simulink model "DigitalTwinMachine"  (R2023b)
settings: Solver=FixedStepAuto  StartTime=0.0  StopTime=0.2  FixedStep=0.001  RelTol=1e-1
undefined symbols (not defined in the file or in its folder): gray
libraries: fl_lib x40, nesl_utility x13, ee_lib x6, batteryecm_lib x1
settings Model: PacingRate=0.022000  Creator=Utente  LastModifiedBy=Utente
settings OptimizationCC: ReuseModelBlockBuffer=off
settings DebuggingCC: ParameterOverflowMsg=none
settings SFSimCC: SimTargetLang=C++

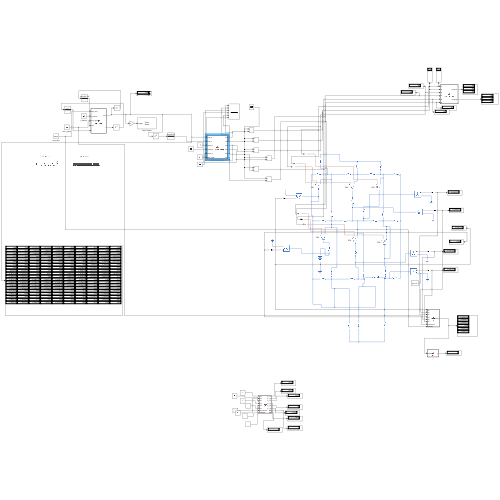
[thumbnail: Simulink's stored preview of the top-level diagram]
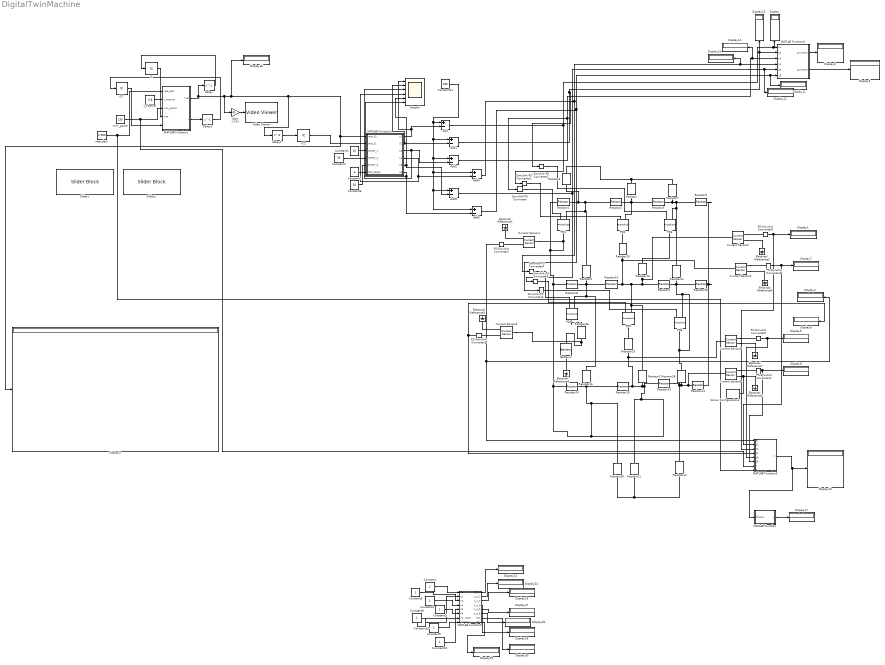
== system DigitalTwinMachine ==
  Add{,1..5} (6 alike) : Sum  Inputs=+-
  Battery1 : batteryecm_lib/Battery  Vnom=12 V  prm_dir=simscape.enum.battery.prm_dir.disabled  R1_dis=2 Ohm  R1_ch=2 Ohm  R1=2 Ohm  prm_AH=simscape.enum.battery.prm_AH.infinite  AH=50 A*hr  V1=11.5 V  AH1=25 A*hr  prm_R2=simscape.enum.battery.prm_R2.disabled  R2=2000 Ohm  Tmeas=298.15 K  charge_measurement_port=simscape.enum.battery.enable.no  prm_dyn=simscape.enum.battery.prm_dyn.off  Rp1=0.005 Ohm  tau1=30 s  Rp2=0.005 Ohm  tau2=30 s  Rp3=0.005 Ohm  tau3=30 s  Rp4=0.005 Ohm  tau4=30 s  Rp5=0.005 Ohm  tau5=30 s  prm_fade=simscape.enum.battery.prm_fade.disabled  N_fade=100  AH_fade=45 A*hr  R1_fade=2.02 Ohm  R1_ch_fade=2.02 Ohm  V1_fade=10.35 V  prm_age=simscape.enum.battery.prm_age.disabled  prm_age_OCV=simscape.enum.battery.prm_age_OCV.OCV  OCV_age=0.9  SOC_age=60  Tmeas_age=298.15 K  delta_time_age_vec=[0] d  temperature_age_vec=[273] K  OCV_scaling_age=2.2134e6  OCV_offset_age=1.632e6  temp_exp_age=0.515833569 V  t_exp_age=0.75  Vnom_T2=12 V  R1_T2=2.2 Ohm  R1_T2_dis=2.2 Ohm  R1_T2_ch=2.2 Ohm  V1_T2=11.4 V  R2_T2=2200 Ohm  Rp1_T2=0.005 Ohm  tau1_T2=30 s  Rp2_T2=0.005 Ohm  tau2_T2=30 s  Rp3_T2=0.005 Ohm  tau3_T2=30 s  Rp4_T2=0.005 Ohm  tau4_T2=30 s  Rp5_T2=0.005 Ohm  tau5_T2=30 s  Tmeas2=273.15 K  thermal_port=simscape.enum.thermaleffects.omit  thermal_mass=30000 J/K  i_specify=off  i_priority=None  i=0 A  i_nominal_specify=off  i_nominal_unit=A  i_nominal_value=1  v_specify=off  v_priority=None  v=0 V  v_nominal_specify=off  v_nominal_unit=V  v_nominal_value=1  charge_specify=off  charge_priority=High  charge=50 A*hr  charge_nominal_specify=off  charge_nominal_unit=A*hr  charge_nominal_value=1  num_cycles_specify=off  num_cycles_priority=High  num_cycles=0  num_cycles_nominal_specify=off  num_cycles_nominal_unit=1  num_cycles_nominal_value=1  temperature_specify=off  temperature_priority=High  temperature=298.15 K  temperature_nominal_specify=off  temperature_nominal_unit=K  temperature_nominal_value=1
  Constant{,3..5,8..10,12} (8 alike) : Constant
  Constant1 : Constant  Value=10
  Constant11 : Constant  Value=185
  Constant2 : Constant  Value=30
  Constant6 : Constant  Value=50
  Constant7 : Constant  Value=6
  Current Sensor{1..6} (6 alike) : fl_lib/Electrical/Electrical Sensors/Current Sensor
  Delay : Delay  DelayLength=1  InitialCondition=0
  Delay1 : Delay  DelayLength=1  InitialCondition=0
  Delay2 : Delay  InitialCondition=0
  Display{,1..17,23..30} (26 alike) : Display
  Electrical Reference{1..7} (7 alike) : fl_lib/Electrical/Electrical Elements/Electrical Reference
  Gain : Gain  Gain=1/255
  IC : InitialCondition  Value=zeros(100,100)
  IC1 : InitialCondition
  IC2 : InitialCondition  Value=zeros(100,100)
  MATLAB Function : MATLAB Function  TreatAsAtomicUnit=on
  MATLAB Function1 : MATLAB Function  TreatAsAtomicUnit=on
  MATLAB Function2 : MATLAB Function  TreatAsAtomicUnit=on
  MATLAB Function3 : MATLAB Function  TreatAsAtomicUnit=on
  MATLAB Function4 : MATLAB Function  TreatAsAtomicUnit=on
  MATLAB Function5 : MATLAB Function  TreatAsAtomicUnit=on
  PD1 : ee_lib/Sensors & Transducers/Photodiode  prmFlux=2  Imeas=25 uA  FluxD=5 W/m^2  G=5e-6 A*m^2/W  prmExp=1  I2=0.1 A  V2=1.3 V  IS=5e-9 A  ec=3  RS=0.1 Ohm  Tmeas=25 degC  C_param=1  CJ=60 pF  CJ0=60 pF  VJ=1 V  Mgrad=0.5  Vvec=[.1, 10, 100] V  Cvec=[45, 3, 6] pF  FC=0.5  T_param=1  IS_T2=2.5e-7 A  I1_T2=0.07 A  V1_T2=1.3 V  Tmeas2=125 degC  EG_param=1  EG=1.11 eV  XTI_param=1  XTI=3  Tdevice=25 degC  i_specify=off  i_priority=None  i=0 A  i_nominal_specify=off  i_nominal_unit=A  i_nominal_value=1  v_specify=off  v_priority=None  v=0 V  v_nominal_specify=off  v_nominal_unit=V  v_nominal_value=1  v_capacitor_specify=off  v_capacitor_priority=High  v_capacitor=0 V  v_capacitor_nominal_specify=off  v_capacitor_nominal_unit=V  v_capacitor_nominal_value=1  thermal_network_parameterization=ee.enum.thermalNetworkTopology.junctionCase  Rth=[0, 10] K/W  Rth_Cauer=[1, 3, 10] K/W  Rth_Foster=[4, 6] K/W  thermal_mass_parameterization=ee.enum.thermalNetwork.timeconstant  thermal_mass=[0, 1] J/K  thermal_mass_Cauer=[1.5, 2, 3] J/K  thermal_mass_Foster=[1.5, 3] J/K  thermal_time_constant=[0, 10] s  thermal_time_constant_Cauer=[1, 3, 10] s  thermal_time_constant_Foster=[6, 18] s  thermal_mass_initial_temperatures=[25, 25] degC  thermal_mass_initial_temperatures_Cauer=[25, 25, 25] degC  steadyState_Foster=simscape.enum.onoff.on  Tvec_initial_Foster=[25, 25, 25, 25] degC
      settings: InternalSimscapePortConfiguration="{\"Bottom\":[],\"Left\":[{\"id\":\"W\",\"label\":\"W\",\"type\":\"input\"},{\"id\":\"p\",\"label\":\"\",\"type\":\"foundation.electrical.electrical\"}],\"Right\":[{\"id\":\"n\",\"label\":\"\",\"type\":\"foundation.electrical.electrical\"}],\"Top\":[]}"
  PD{2..3,5..6} (4 alike) : ee_lib/Sensors & Transducers/Photodiode  prmFlux=1  Imeas=25 uA  FluxD=5 W/m^2  G=5e-6 A*m^2/W  prmExp=1  I2=0.1 A  V2=1.3 V  IS=5e-9 A  ec=3  RS=0.1 Ohm  Tmeas=25 degC  C_param=1  CJ=60 pF  CJ0=60 pF  VJ=1 V  Mgrad=0.5  Vvec=[.1, 10, 100] V  Cvec=[45, 3, 6] pF  FC=0.5  T_param=1  IS_T2=2.5e-7 A  I1_T2=0.07 A  V1_T2=1.3 V  Tmeas2=125 degC  EG_param=1  EG=1.11 eV  XTI_param=1  XTI=3  Tdevice=25 degC  i_specify=off  i_priority=None  i=0 A  i_nominal_specify=off  i_nominal_unit=A  i_nominal_value=1  v_specify=off  v_priority=None  v=0 V  v_nominal_specify=off  v_nominal_unit=V  v_nominal_value=1  v_capacitor_specify=off  v_capacitor_priority=High  v_capacitor=0 V  v_capacitor_nominal_specify=off  v_capacitor_nominal_unit=V  v_capacitor_nominal_value=1  thermal_network_parameterization=ee.enum.thermalNetworkTopology.junctionCase  Rth=[0, 10] K/W  Rth_Cauer=[1, 3, 10] K/W  Rth_Foster=[4, 6] K/W  thermal_mass_parameterization=ee.enum.thermalNetwork.timeconstant  thermal_mass=[0, 1] J/K  thermal_mass_Cauer=[1.5, 2, 3] J/K  thermal_mass_Foster=[1.5, 3] J/K  thermal_time_constant=[0, 10] s  thermal_time_constant_Cauer=[1, 3, 10] s  thermal_time_constant_Foster=[6, 18] s  thermal_mass_initial_temperatures=[25, 25] degC  thermal_mass_initial_temperatures_Cauer=[25, 25, 25] degC  steadyState_Foster=simscape.enum.onoff.on  Tvec_initial_Foster=[25, 25, 25, 25] degC
      settings: InternalSimscapePortConfiguration="{\"Bottom\":[],\"Left\":[{\"id\":\"W\",\"label\":\"W\",\"type\":\"input\"},{\"id\":\"p\",\"label\":\"\",\"type\":\"foundation.electrical.electrical\"}],\"Right\":[{\"id\":\"n\",\"label\":\"\",\"type\":\"foundation.electrical.electrical\"}],\"Top\":[]}"
  PD4 : ee_lib/Sensors & Transducers/Photodiode  prmFlux=1  Imeas=25 uA  FluxD=5 W/m^2  G=5e-6 A*m^2/W  prmExp=1  I2=1 A  V2=10 V  IS=5e-9 A  ec=3  RS=0.1 Ohm  Tmeas=25 degC  C_param=1  CJ=60 pF  CJ0=60 pF  VJ=1 V  Mgrad=0.5  Vvec=[.1, 10, 100] V  Cvec=[45, 3, 6] pF  FC=0.5  T_param=1  IS_T2=2.5e-7 A  I1_T2=0.07 A  V1_T2=1.3 V  Tmeas2=125 degC  EG_param=1  EG=1.11 eV  XTI_param=1  XTI=3  Tdevice=25 degC  i_specify=off  i_priority=None  i=0 A  i_nominal_specify=off  i_nominal_unit=A  i_nominal_value=1  v_specify=off  v_priority=None  v=0 V  v_nominal_specify=off  v_nominal_unit=V  v_nominal_value=1  v_capacitor_specify=off  v_capacitor_priority=High  v_capacitor=0 V  v_capacitor_nominal_specify=off  v_capacitor_nominal_unit=V  v_capacitor_nominal_value=1  thermal_network_parameterization=ee.enum.thermalNetworkTopology.junctionCase  Rth=[0, 10] K/W  Rth_Cauer=[1, 3, 10] K/W  Rth_Foster=[4, 6] K/W  thermal_mass_parameterization=ee.enum.thermalNetwork.timeconstant  thermal_mass=[0, 1] J/K  thermal_mass_Cauer=[1.5, 2, 3] J/K  thermal_mass_Foster=[1.5, 3] J/K  thermal_time_constant=[0, 10] s  thermal_time_constant_Cauer=[1, 3, 10] s  thermal_time_constant_Foster=[6, 18] s  thermal_mass_initial_temperatures=[25, 25] degC  thermal_mass_initial_temperatures_Cauer=[25, 25, 25] degC  steadyState_Foster=simscape.enum.onoff.on  Tvec_initial_Foster=[25, 25, 25, 25] degC
      settings: InternalSimscapePortConfiguration="{\"Bottom\":[],\"Left\":[{\"id\":\"W\",\"label\":\"W\",\"type\":\"input\"},{\"id\":\"p\",\"label\":\"\",\"type\":\"foundation.electrical.electrical\"}],\"Right\":[{\"id\":\"n\",\"label\":\"\",\"type\":\"foundation.electrical.electrical\"}],\"Top\":[]}"
  PS-Simulink Converter{1..6} (6 alike) : nesl_utility/PS-Simulink Converter  PhysicalDomain=network_engine_domain  SubClassName=ps_output  LeftPortType=input  RightPortType=output  PseudoPeriodic=off  Frequencies=[]  VectorFormat=inherit  Unit=inherit  AffineConversion=off
  Resistor{,1..25} (26 alike) : fl_lib/Electrical/Electrical Elements/Resistor  R=1 Ohm  i_specify=off  i_priority=None  i=0 A  i_nominal_specify=off  i_nominal_unit=A  i_nominal_value=1  v_specify=off  v_priority=None  v=0 V  v_nominal_specify=off  v_nominal_unit=V  v_nominal_value=1
  Resistor26 : fl_lib/Electrical/Electrical Elements/Resistor  R=1.3 Ohm  i_specify=off  i_priority=None  i=0 A  i_nominal_specify=off  i_nominal_unit=A  i_nominal_value=1  v_specify=off  v_priority=None  v=0 V  v_nominal_specify=off  v_nominal_unit=V  v_nominal_value=1
  Scope5 : Scope  NumInputPorts=6
  Simulink-PS Converter{,1..5} (6 alike) : nesl_utility/Simulink-PS Converter  PhysicalDomain=network_engine_domain  SubClassName=ps_input  LeftPortType=input  RightPortType=output  PseudoPeriodic=off  Frequencies=[]  NoiseDistribution=none  NoiseParameters=[]  Unit=1  AffineConversion=off  FilteringAndDerivatives=provide  SimscapeFilterOrder=1  InputFilterTimeConstant=0.001  UdotUserProvided=0
  Slider1 : SliderBlock  ScaleMin=0.1  ScaleMax=1
  Slider2 : SliderBlock  ScaleMin=1  ScaleMax=150  TickInterval=1
  Solver Configuration3 : nesl_utility/Solver Configuration  PhysicalDomain=network_engine_domain  SubClassName=solver  LeftPortType=input  RightPortType=generic  Tones=[]  Harmonics=[]  SimulateNoise=off  Profile=off  UseLocalSampling=off  EnableSwitchedLinearOptims=on  FrequencyDomain=off  UseCCode=off  RelTol=0.001  AbsTol=0.001  MinStep=1e-09  ToWorkspace=off  RevertToSquareIcSolve=off  NumHomotopyIterations=100  PhasorMode=off  PhasorModeNumHarmonics=1  ConsistencySolver=NEWTON_XTOL_AFTER_FTOL  IndexReductionMethod=DerivativeReplacement  DoDC=off  ResidualTolerance=1e-09  ConsistencyTolSource=GLOBAL  ConsistencyAbsTol=0.001  ConsistencyRelTol=0.001  ConsistencyTolFactor=0.001  UseLocalSolver=off  LocalSolverChoice=NE_BACKWARD_EULER_ADVANCER  ResolveIndetEquations=on  FunctionEvalNumThread=1  LocalSolverSampleTime=0.001  DoFixedCost=off  MaxNonlinIter=3  MaxModeIter=2  ComputeImpulses=off  ImpulseIterations=2  LinearAlgebra=auto  LinearAlgebraNumThread=0  EquationFormulation=NE_TIME_EF  DelaysMemoryBudget=1024  AutomaticFiltering=on  FilteringTimeConstant=0.001  PartitionStorageMethod=AS_NEEDED  PartitionMemoryBudget=1024  PartitionMethod=ROBUST  MultibodyUseLocalSolver=off  MultibodyLocalSolverChoice=ODE1  MultibodyLocalSolverSampleTime=0.001
  Video Viewer : VideoViewer  colormapValue=gray(256)  FigPos=[1 814 1536 716]
  num_gocce : Constant  Value=135  OutDataTypeStr=int8
  rate_decr : Constant  Value=0.900
  t_interval : Constant  Value=0.8
  wires:
  Constant11/1 -> Add5/1, Add3/1, Add4/1, Add2/1, Add1/1, Add/1
  MATLAB Function2/2(s2) -> Scope5/2, Add1/2
  MATLAB Function2/3(s3) -> Scope5/3, Add2/2
  MATLAB Function2/1(s1) -> Scope5/1, Add/2
  MATLAB Function4/1(arrmem1) -> Display4/1
  MATLAB Function2/4(s4) -> Scope5/4, Add4/2
  MATLAB Function2/5(s5) -> Scope5/5, Add5/2
  MATLAB Function2/6(s6) -> Scope5/6, Add3/2
  rate_decr/1 -> MATLAB Function3/8(rateDecr), MATLAB Function1/1(rate_decr)
  num_gocce/1 -> MATLAB Function3/7(numGocce), MATLAB Function1/3(num_gocce)
  t_interval/1 -> MATLAB Function1/2(t_interval)
  MATLAB Function1/1(mat) -> Display16/1, Display3/1, MATLAB Function2/1(mat_t0), Delay2/1, Gain/1, Delay/1
  IC/1 -> MATLAB Function1/4("mat ")
  Delay/1 -> IC/1
  Constant1/1 -> MATLAB Function2/3(center_1)
  Constant2/1 -> MATLAB Function2/4(center_2)
  Constant6/1 -> MATLAB Function2/5(center_3)
  Constant7/1 -> MATLAB Function2/6(half_height)
  MATLAB Function1/2(t) -> Delay1/1
  Delay1/1 -> IC1/1
  IC1/1 -> MATLAB Function1/5("t ")
  Gain/1 -> Video Viewer/1
  Delay2/1 -> IC2/1
  IC2/1 -> MATLAB Function2/2(mat_t1)
  MATLAB Function4/2(arrmem2) -> Display5/1
  Add/1 -> Display/1, MATLAB Function4/1(s1), Simulink-PS Converter1/1
  Add1/1 -> Display15/1, MATLAB Function4/2(s2), Simulink-PS Converter2/1
  Add2/1 -> Display14/1, MATLAB Function4/3(s3), Simulink-PS Converter/1
  Add4/1 -> Simulink-PS Converter4/1, Display13/1, MATLAB Function4/4(s4)
  Add5/1 -> Display12/1, MATLAB Function4/5(s5), Simulink-PS Converter5/1
  Add3/1 -> Display11/1, MATLAB Function4/6(s6), Simulink-PS Converter3/1
  PS-Simulink Converter6/1 -> MATLAB Function3/3(s3), Display1/1
  PS-Simulink Converter1/1 -> MATLAB Function3/1(s1), Display2/1
  PS-Simulink Converter2/1 -> MATLAB Function3/4(s4), Display6/1
  PS-Simulink Converter3/1 -> MATLAB Function3/2(s2), Display7/1
  PS-Simulink Converter4/1 -> MATLAB Function3/6(s6), Display8/1
  PS-Simulink Converter5/1 -> MATLAB Function3/5(s5), Display9/1
  MATLAB Function3/1(outputArray) -> MATLAB Function/1(listSum), Display10/1
  MATLAB Function5/6(s_o_6) -> Display28/1
  MATLAB Function5/3(s_o_3) -> Display25/1
  MATLAB Function5/4(s_o_4) -> Display26/1
  MATLAB Function5/2(s_o_2) -> Display24/1
  MATLAB Function5/1(s_o_1) -> Display23/1
  MATLAB Function5/8(RD) -> Display29/1
  MATLAB Function5/5(s_o_5) -> Display27/1
  MATLAB Function5/7(NG) -> Display30/1
  Constant/1 -> MATLAB Function5/1(s1)
  Constant9/1 -> MATLAB Function5/8(rateDecr)
  Constant8/1 -> MATLAB Function5/7(numGocce)
  Constant5/1 -> MATLAB Function5/6(s6)
  Constant4/1 -> MATLAB Function5/4(s4)
  Constant3/1 -> MATLAB Function5/3(s3)
  Constant12/1 -> MATLAB Function5/5(s5)
  Constant10/1 -> MATLAB Function5/2(s2)
  MATLAB Function/1(y) -> Display17/1
  connections:
  PD2/LConn2 -- Resistor3/LConn1 -- Resistor/RConn1 -- Resistor2/RConn1
  Current Sensor4/LConn1 -- Resistor19/RConn1 -- Resistor14/LConn1 -- Current Sensor2/LConn1 -- Resistor13/RConn1 -- Resistor4/LConn1 -- Resistor17/LConn1 -- PD5/LConn2
  Resistor2/LConn1 -- Resistor1/RConn1 -- Resistor6/RConn1 -- Resistor5/LConn1 -- PD1/LConn2
  Electrical Reference4/LConn1 -- Battery1/RConn1
  Resistor10/LConn1 -- Resistor4/RConn1 -- Resistor12/RConn1 -- PD6/RConn1 -- Resistor18/LConn1 -- PD6/LConn2
  Resistor16/LConn1 -- PD4/LConn2 -- Resistor14/RConn1 -- Resistor5/RConn1 -- Resistor8/RConn1
  Resistor7/LConn1 -- Resistor6/LConn1 -- Resistor/LConn1
  Resistor7/RConn1 -- Resistor3/RConn1 -- Resistor9/RConn1 -- Resistor12/LConn1 -- PD3/LConn2
  Resistor18/RConn1 -- Current Sensor5/LConn1 -- Resistor11/LConn1 -- Resistor23/RConn1 -- Resistor22/LConn1
  Resistor26/RConn1 -- Current Sensor3/LConn1 -- Battery1/LConn1
  Resistor21/LConn1 -- Resistor16/RConn1 -- Resistor24/RConn1 -- Resistor15/LConn1 -- Resistor20/LConn1 -- Resistor24/LConn1 -- PD1/RConn1 -- Current Sensor1/LConn1 -- Resistor1/LConn1 -- Resistor8/LConn1 -- Resistor23/LConn1 -- Resistor17/RConn1 -- Current Sensor6/LConn1 -- Resistor25/RConn1 -- Resistor15/RConn1
  Resistor10/RConn1 -- Resistor9/LConn1 -- Resistor11/RConn1
  Simulink-PS Converter/RConn1 -- PD1/LConn1
  Simulink-PS Converter1/RConn1 -- PD2/LConn1
  Simulink-PS Converter2/RConn1 -- PD3/LConn1
  Simulink-PS Converter3/RConn1 -- PD6/LConn1
  Simulink-PS Converter5/RConn1 -- PD5/LConn1
  Simulink-PS Converter4/RConn1 -- PD4/LConn1
  Current Sensor2/RConn2 -- Electrical Reference2/LConn1
  Current Sensor2/RConn1 -- PS-Simulink Converter6/LConn1
  PD3/RConn1 -- Resistor13/LConn1
  Current Sensor1/RConn1 -- PS-Simulink Converter1/LConn1
  Current Sensor1/RConn2 -- Electrical Reference1/LConn1
  Current Sensor3/RConn1 -- PS-Simulink Converter2/LConn1
  Current Sensor3/RConn2 -- Electrical Reference3/LConn1
  Resistor19/LConn1 -- PD2/RConn1
  Current Sensor4/RConn1 -- PS-Simulink Converter3/LConn1
  Current Sensor4/RConn2 -- Electrical Reference5/LConn1
  Resistor20/RConn1 -- Resistor21/RConn1 -- Resistor22/RConn1
  Current Sensor5/RConn1 -- PS-Simulink Converter4/LConn1
  Current Sensor5/RConn2 -- Solver Configuration3/RConn1 -- Electrical Reference6/LConn1
  PD5/RConn1 -- Resistor25/LConn1
  Current Sensor6/RConn2 -- Electrical Reference7/LConn1
  Current Sensor6/RConn1 -- PS-Simulink Converter5/LConn1
  PD4/RConn1 -- Resistor26/LConn1

== matlab function DigitalTwinMachine/MATLAB Function ==
  data: listSum input; y output
function y = fcn(listSum)

input_List = listSum;
coder.extrinsic('writematrix','readmatrix')
%dlmwrite('firstCsv.txt',input_List,'-append');
writematrix(input_List,"csv53.txt",'WriteMode','append');
y = 1;
%y = readmatrix("fifthCsv.txt");
class(y)

== matlab function DigitalTwinMachine/MATLAB Function1 ==
  settings: updateMethod=DISCRETE
  data: rate_decr input; t_interval input; num_gocce input; mat input; mat output; t input; t output
function [mat,t] = rain_mat(rate_decr,t_interval,num_gocce,mat,t)
    %z = zeros(side,side,t_max);
    %for t = 1:t_max
    mat(mat ~= 0) = mat(mat ~= 0) - rate_decr * 255;
    if rem(t,t_interval) == 0
        mat = create_mat(mat,100,rate_decr,num_gocce);
    end
    t = t+1;
        
        %img = image(mat)
        %z(:,:,t) = mat;
    %end
end

== matlab function DigitalTwinMachine/MATLAB Function5 ==
  settings: updateMethod=DISCRETE
  data: s1 input; s_o_1 output; s2 input; s3 input; s4 input; s5 input; s6 input; s_o_2 output; s_o_3 output; s_o_4 output; s_o_5 output; s_o_6 output; numGocce input; rateDecr input; NG output; RD output
function [s_o_1,s_o_2,s_o_3,s_o_4,s_o_5,s_o_6,NG,RD]= fcn(s1,s2,s3,s4,s5,s6, numGocce,rateDecr)

R1F = 0.1+1.9*rand(1,1);
R4F = 0.1+5.0*rand(1,1);
R5F = 0.1+101.0*rand(1,1);
R2F = 0.1+2.9*rand(1,1);
R3F = 0.1+3.9*rand(1,1);

R1D = 0.1+98.0*rand(1,1);
R2D = 0.1+108.0*rand(1,1);
R3D = 0.1+115.0*rand(1,1);
R4D = 0.1+68.0*rand(1,1);
R5D = 0.1+151.0*rand(1,1);
R6 = 0.1+69.0*rand(1,1);

NG = numGocce;
RD = rateDecr;

if(numGocce > 45.0 && numGocce <= 90.0) && (rateDecr > 0.25 && rateDecr <= 0.5)

    if s1 > 92.0 
        s_o_1 = 92.0 - R1F;

    elseif s1 < 90.0  
        s_o_1 = 90.0 + R1F;

    else
        s_o_1 = s1;

    end

    if s2 > 98.0 
        s_o_2 = 98.0 - R2F;

    elseif s2 < 95.0  
        s_o_2 = 95.0 + R2F;

    else
        s_o_2 = s2;

    end

    if s3 > 101.0 
        s_o_3 = 101.0 - R3F;

    elseif s3 < 97.0  
        s_o_3 = 97.0 + R3F;

    else
        s_o_3 = s3;

    end
    



    if s4 < 179.0 
        s_o_4 = 179.0 + R4F;

    elseif s4 > 184.0  
        s_o_4 = 184.0 - R4F;

    else
        s_o_4 = s4;

    end

    if s5 < 96.0 
        s_o_5 = 96.0 + R5F;

    elseif s5 > 197.0  
        s_o_5 = 197.0 - R5F;

    else
        s_o_5 = s5;

    end

    if s6 > 177.0 
        s_o_6 = 177.0 - R1F;

    elseif s6 < 175.0  
        s_o_6 = 175.0 + R1F;

    else
        s_o_6 = s6;

    end

else

    if s2 > 113.0 
        s_o_2 = 113.0 - R2D;

    elseif s2 < 5.0  
        s_o_2 = 5.0 + R2D;

    else
        s_o_2 = s2;

    end
    
    if s3 > 121.0 
        s_o_3 = 121.0 - R3D;

    elseif s3 < 6.0  
        s_o_3 = 6.0 + R3D;

    else
        s_o_3 = s3;

    end

    if s1 > 103.0 
        s_o_1 = 103.0 - R1D;

    elseif s1 < 5.0  
        s_o_1 = 5.0 + R1D;

    else
        s_o_1 = s1;

    end


    if s4 < 4.0 
        s_o_4 = 72.0 + R4D;

    elseif s4 > 72.0  
        s_o_4 = 4.0 - R4D;

    else
        s_o_4 = s4;

    end

    if s5 < 5.0 
        s_o_5 = 5.0 + R5D;

    elseif s5 > 156.0  
        s_o_5 = 156.0 - R5D;

    else
        s_o_5 = s5;

    end

    if s6 > 73.0 
        s_o_6 = 73.0 - R6;

    elseif s6 < 4.0  
        s_o_6 = 4.0 + R6;

    else
        s_o_6 = s6;

    end

end



end

== matlab function DigitalTwinMachine/MATLAB Function2 ==
  data: s1 output; mat_t0 input; mat_t1 input; s2 output; s3 output; s4 output; s5 output; s6 output; center_1 input; center_2 input; center_3 input; half_height input
function [s1,s2,s3,s4,s5,s6] = get_params_diode(mat_t0,mat_t1,center_1,center_2,center_3,half_height)
    acc1 = 0;
    acc2 = 0;
    acc3 = 0;
    acc4 = 0;
    acc5 = 0;
    acc6 = 0;
    minVal0 = [88,9,7,6,6];
    maxVal0 = [90,187,176,136,133];
    minVal1 = [79,12,9,7,6];
    maxVal1 = [139,118,214,140,83];
    minVal2 = [97,10,8,6,6];
    maxVal2 = [100,155,200,152,128];
    minVal3 = [194,8,7,5,6];
    maxVal3 = [197,258,351,230,235];
    minVal4 = [203,11,8,6,6];
    maxVal4 = [213,244,271,223,214];
    minVal5 = [185,8,7,6,5];
    maxVal5 = [190,258,233,168,214];
    for i = 1:size(mat_t0,1)
        for i_2 = center_1-half_height:center_1+half_height
            if mat_t0(i,i_2) >= 127.500
                acc1 = acc1 + 1;
            end
        end
    end

    for j = 1:size(mat_t0,1)
        for j_2 = center_2-half_height:center_2+half_height
            if mat_t0(j,j_2) >= 127.500
                acc2 = acc2 + 1;
            end
        end
    end

    for k = 1:size(mat_t0,1)
        for k_2 = center_3-half_height:center_3+half_height
            if mat_t0(k,k_2) >= 127.500
                acc3 = acc3 + 1;
            end
        end
    end

    for i = 1:size(mat_t1,1)
        for i_2 = center_1-half_height:center_1+half_height
            if mat_t1(i,i_2) >= 127.500
                acc4 = acc4 + 1;
            end
        end
    end

    for j = 1:size(mat_t1,1)
        for j_2 = center_2-half_height:center_2+half_height
            if mat_t1(j,j_2) >= 127.500
                acc5 = acc5 + 1;
            end
        end
    end

    for k = 1:size(mat_t1,1)
        for k_2 = center_3-half_height:center_3+half_height
            if mat_t1(k,k_2) >= 127.500
                acc6 = acc6 + 1;
            end
        end
    end
    s1 = acc1;
    s2 = acc2;
    s3 = acc3;
    s4 = acc4;
    s5 = acc5;
    s6 = acc6;



end

== matlab function DigitalTwinMachine/MATLAB Function3 ==
  settings: updateMethod=DISCRETE
  data: s1 input; outputArray output; s2 input; s3 input; s4 input; s5 input; s6 input; numGocce input; rateDecr input
function outputArray = fcn(s1,s2,s3,s4,s5,s6, numGocce, rateDecr)

minVal0 = [88,9,7,6,6];
maxVal0 = [90,187,176,136,133];
minVal1 = [79,12,9,7,6];
maxVal1 = [139,118,214,140,83];
minVal2 = [97,10,8,6,6];
maxVal2 = [100,155,200,152,128];
minVal3 = [194,8,7,5,6];
maxVal3 = [197,258,351,230,235];
minVal4 = [203,11,8,6,6];
maxVal4 = [213,244,271,223,214];
minVal5 = [185,8,7,6,5];
maxVal5 = [190,258,233,168,214];
indexClasses = [0,1,2,3,4]
value_rain = 4
value_rate = 4

outputArray = [s1,s2,s3,s4,s5,s6];


switch numGocce

    case (numGocce >= 0 && numGocce <= 30) && (rateDecr >= 0.0 && rateDecr <= 0.2)
        value_rain = indexClasses(1);
        value_rate = indexClasses(1);

    case ((numGocce > 30 && numGocce <= 60) && (rateDecr > 0.2 && rateDecr <= 0.4)) || ((numGocce >= 0 && numGocce <= 30) && (rateDecr > 0.4 && rateDecr <= 0.6)) || ((numGocce > 60 && numGocce <= 90) && (rateDecr >= 0.0 && rateDecr <= 0.2))
        value_rain = indexClasses(2);
        value_rate = indexClasses(2);
    
    case ((numGocce > 60 && numGocce <= 90) && (rateDecr > 0.4 && rateDecr <= 0.6)) || ((numGocce > 30 && numGocce <= 60) && (rateDecr > 0.6 && rateDecr <= 0.8)) || ((numGocce > 90 && numGocce <= 120) && (rateDecr > 0.2 && rateDecr <= 0.4)) || ((numGocce >= 0 && numGocce <= 30) && (rateDecr > 0.8 && rateDecr <= 1.0)) || ((numGocce > 120 && numGocce <= 150) && (rateDecr >= 0.0 && rateDecr <= 0.2))
        value_rain = indexClasses(3);
        value_rate = indexClasses(3);

    case ((numGocce > 90 && numGocce <= 120) && (rateDecr > 0.6 && rateDecr <= 0.8)) || ((numGocce > 60 && numGocce <= 90) && (rateDecr > 0.8 && rateDecr <= 1.0)) || ((numGocce > 120 && numGocce <= 150) && (rateDecr > 0.4 && rateDecr <= 0.6))
        value_rain = indexClasses(4);
        value_rate = indexClasses(4);

    case (numGocce > 120 && numGocce <= 150) && (rateDecr > 0.8 && rateDecr <= 1.0)
        value_rain = indexClasses(5);
        value_rate = indexClasses(5);

end

switch value_rain

    case value_rain == 0 && value_rate == 0
        if outputArray(1) < minVal0(1) || outputArray(1) > maxVal0(1)
            outputArray(1) = 89;

        end

        if outputArray(2) < minVal1(1) || outputArray(2) > maxVal1(1)
            outputArray(2) = -30+30*rand(1,1);

        end

        if outputArray(3) < minVal2(1) || outputArray(3) > maxVal2(1)
            outputArray(3) = -1+1*rand(1,1);

        end

        if outputArray(4) < minVal3(1) || outputArray(4) > maxVal3(1)
            outputArray(4) = -1+1*rand(1,1);

        end

        if outputArray(5) < minVal4(1) || outputArray(5) > maxVal4(1)
            outputArray(5) = -5+5*rand(1,1);

        end

        if outputArray(6) < minVal5(1) || outputArray(6) > maxVal5(1)
            outputArray(6) = -2+2*rand(1,1);

        end

    case value_rain == 1 && value_rate == 1
        if outputArray(1) < minVal0(2) || outputArray(1) > maxVal0(2)
            outputArray(1) = -85+85*rand(1,1);

        end

        if outputArray(2) < minVal1(2) || outputArray(2) > maxVal1(2)
            outputArray(2) = -53+53*rand(1,1);

        end

        if outputArray(3) < minVal2(2) || outputArray(3) > maxVal2(2)
            outputArray(3) = -70+70*rand(1,1);

        end

        if outputArray(4) < minVal3(2) || outputArray(4) > maxVal3(2)
            outputArray(4) = -125+125*rand(1,1);

        end

        if outputArray(5) < minVal4(2) || outputArray(5) > maxVal4(2)
            outputArray(5) = -115+115*rand(1,1);

        end

        if outputArray(6) < minVal5(2) || outputArray(6) > maxVal5(2)
            outputArray(6) = -125+125*rand(1,1);

        end

    case value_rain == 2 && value_rate == 2
        if outputArray(1) < minVal0(3) || outputArray(1) > maxVal0(3)
            outputArray(1) = -85+85*rand(1,1);

        end

        if outputArray(2) < minVal1(3) || outputArray(2) > maxVal1(3)
            outputArray(2) = -102+102*rand(1,1);

        end

        if outputArray(3) < minVal2(3) || outputArray(3) > maxVal2(3)
            outputArray(3) = -95+95*rand(1,1);

        end

        if outputArray(4) < minVal3(3) || outputArray(4) > maxVal3(3)
            outputArray(4) = -167+167*rand(1,1);

        end

        if outputArray(5) < minVal4(3) || outputArray(5) > maxVal4(3)
            outputArray(5) = -130+130*rand(1,1);

        end

        if outputArray(6) < minVal5(3) || outputArray(6) > maxVal5(3)
            outputArray(6) = -113+113*rand(1,1);

        end

    case value_rain == 3 && value_rate == 3
        if outputArray(1) < minVal0(4) || outputArray(1) > maxVal0(4)
            outputArray(1) = -165+165*rand(1,1);

        end

        if outputArray(2) < minVal1(4) || outputArray(2) > maxVal1(4)
            outputArray(2) = -66+66*rand(1,1);

        end

        if outputArray(3) < minVal2(4) || outputArray(3) > maxVal2(4)
            outputArray(3) = -73+73*rand(1,1);

        end

        if outputArray(4) < minVal3(4) || outputArray(4) > maxVal3(4)
            outputArray(4) = -112+112*rand(1,1);

        end

        if outputArray(5) < minVal4(4) || outputArray(5) > maxVal4(4)
            outputArray(5) = -108+108*rand(1,1);

        end

        if outputArray(6) < minVal5(4) || outputArray(6) > maxVal5(4)
            outputArray(6) = -81+81*rand(1,1);

        end

    case value_rain == 4 && value_rate == 4
        if outputArray(1) < minVal0(5) || outputArray(1) > maxVal0(5)
            outputArray(1) = -63+63*rand(1,1);

        end

        if outputArray(2) < minVal1(5) || outputArray(2) > maxVal1(5)
            outputArray(2) = -38+38*rand(1,1);

        end

        if outputArray(3) < minVal2(5) || outputArray(3) > maxVal2(5)
            outputArray(3) = -61+61*rand(1,1);

        end

        if outputArray(4) < minVal3(5) || outputArray(4) > maxVal3(5)
            outputArray(4) = -114+114*rand(1,1);

        end

        if outputArray(5) < minVal4(5) || outputArray(5) > maxVal4(5)
            outputArray(5) = -104+104*rand(1,1);

        end

        if outputArray(6) < minVal5(5) || outputArray(6) > maxVal5(5)
            outputArray(6) = -104+104*rand(1,1);

        end

end

end

== matlab function DigitalTwinMachine/MATLAB Function4 ==
  data: s1 input; arrmem1 output; s2 input; s3 input; s4 input; s5 input; s6 input; arrmem2 output
function [arrmem1,arrmem2]  = mem_visualize(s1,s2,s3,s4,s5,s6)

    arrmem1 = [s1,s2,s3]
    %arrmem2 = [s4,s5,s6]
    arrmem2 = [s1,s2,s3]
   
end
